simulink model "PWM_SPWM"  (R2024b)
settings: Solver=VariableStepAuto  StartTime=0.0  StopTime=10.0  RelTol=1e-3
libraries: simulink x2
settings Model: Creator=sanja  LastModifiedBy=sanja

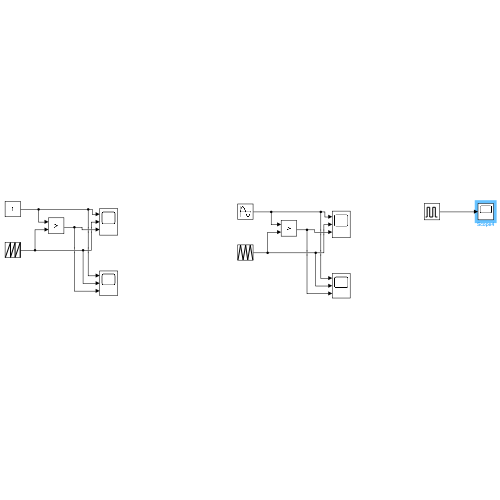
[thumbnail: Simulink's stored preview of the top-level diagram]
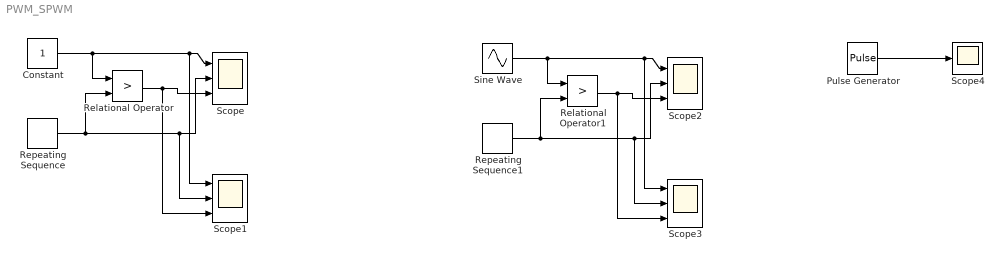
== system PWM_SPWM ==
  Constant : Constant
  Pulse Generator : DiscretePulseGenerator  PulseType=Time based  Period=5  PulseWidth=50
  Relational Operator : RelationalOperator  Operator=>  OutDataTypeStr=boolean  RndMeth=Simplest  InputSameDT=off
  Relational Operator1 : RelationalOperator  Operator=>  OutDataTypeStr=boolean  RndMeth=Simplest  InputSameDT=off
  Repeating Sequence : simulink/Sources/Repeating Sequence  rep_seq_t=[0 2]  rep_seq_y=[0 2]
  Repeating Sequence1 : simulink/Sources/Repeating Sequence  rep_seq_t=[0 0.5 1]  rep_seq_y=[0 2 0]
  Scope{,1..3} (4 alike) : Scope  NumInputPorts=3
  Scope4 : Scope
  Sine Wave : Sin  Frequency=0.5  SampleTime=0
  wires:
  Constant/1 -> Scope1/1, Scope/1, Relational Operator/1
  Repeating Sequence/1 -> Scope1/2, Scope/2, Relational Operator/2
  Relational Operator/1 -> Scope1/3, Scope/3
  Repeating Sequence1/1 -> Scope3/2, Scope2/2, Relational Operator1/2
  Sine Wave/1 -> Scope3/1, Scope2/1, Relational Operator1/1
  Relational Operator1/1 -> Scope3/3, Scope2/3
  Pulse Generator/1 -> Scope4/1
